simulink library "INT_Rail_SetPointAddCor"  (R2016b)
settings: Solver=VariableStepAuto  StartTime=0.0  StopTime=10.0  RelTol=1e-3
settings Model: Creator=Administrator  LastModifiedBy=Administrator

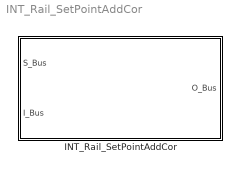
== system INT_Rail_SetPointAddCor ==
  INT_Rail_SetPointAddCor : Subsystem

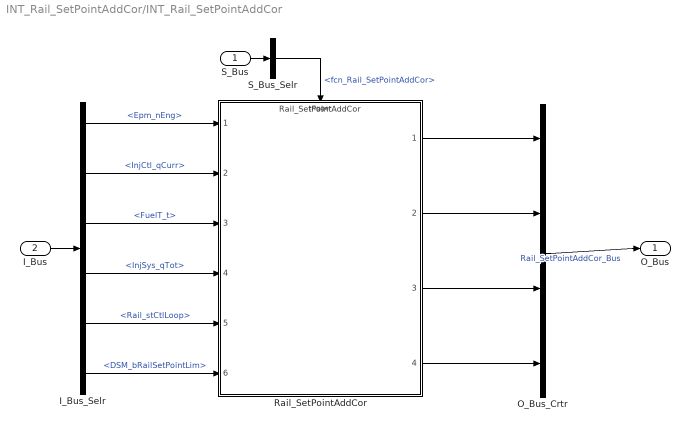
== system INT_Rail_SetPointAddCor/INT_Rail_SetPointAddCor ==
  S_Bus : Inport
  I_Bus : Inport  Port=2
  I_Bus_Selr : BusSelector  OutputSignals=Epm_nEng,InjCtl_qCurr,FuelT_t,InjSys_qTot,Rail_stCtlLoop,DSM_bRailSetPointLim
  O_Bus_Crtr : BusCreator  Inputs=4
  Rail_SetPointAddCor : ModelReference  ModelNameDialog=Rail_SetPointAddCor  SimulationMode=Normal  ModelReferenceVersion=1.10  TriggerPortName=function  TriggerPortTriggerType=function-call  TriggerPortStatesWhenEnabling=held
  S_Bus_Selr : BusSelector  OutputSignals=fcn_Rail_SetPointAddCor
  O_Bus : Outport
  wires:
  S_Bus_Selr/1 -> Rail_SetPointAddCor/Trigger  "<fcn_Rail_SetPointAddCor>"
  S_Bus/1 -> S_Bus_Selr/1
  I_Bus/1 -> I_Bus_Selr/1
  I_Bus_Selr/1 -> Rail_SetPointAddCor/1  "<Epm_nEng>"
  I_Bus_Selr/2 -> Rail_SetPointAddCor/2  "<InjCtl_qCurr>"
  I_Bus_Selr/3 -> Rail_SetPointAddCor/3  "<FuelT_t>"
  I_Bus_Selr/4 -> Rail_SetPointAddCor/4  "<InjSys_qTot>"
  I_Bus_Selr/5 -> Rail_SetPointAddCor/5  "<Rail_stCtlLoop>"
  I_Bus_Selr/6 -> Rail_SetPointAddCor/6  "<DSM_bRailSetPointLim>"
  O_Bus_Crtr/1 -> O_Bus/1  "Rail_SetPointAddCor_Bus"
  Rail_SetPointAddCor/1 -> O_Bus_Crtr/1
  Rail_SetPointAddCor/2 -> O_Bus_Crtr/2
  Rail_SetPointAddCor/3 -> O_Bus_Crtr/3
  Rail_SetPointAddCor/4 -> O_Bus_Crtr/4
